simulink model "Book6331"  (R2019b)
settings: Solver=ode4  StartTime=0.0  StopTime=10.0  FixedStep=0.001  RelTol=1e-3
settings Model: Creator=user  LastModifiedBy=user

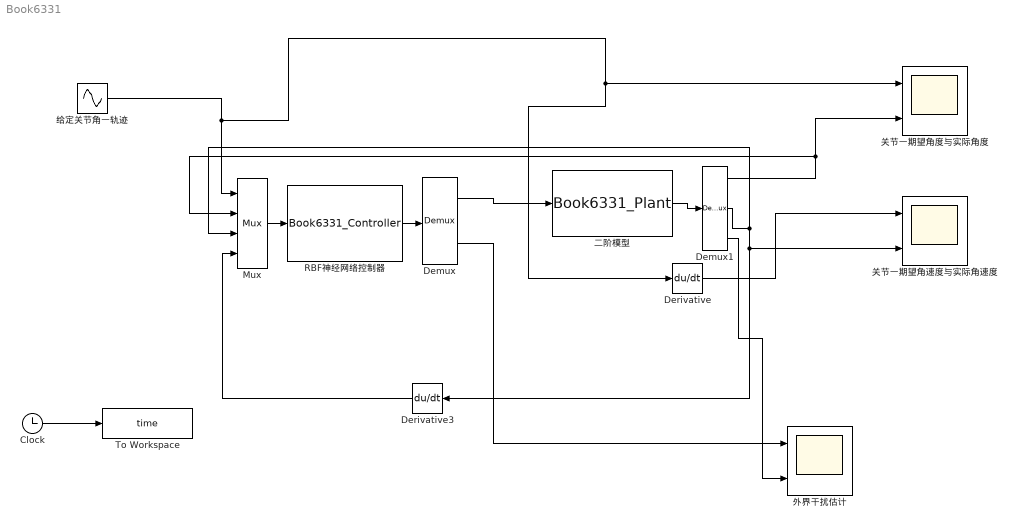
== system Book6331 ==
  Clock : Clock
  Demux : Demux  Outputs=2
  Demux1 : Demux  Outputs=3
  Derivative : Derivative
  Derivative3 : Derivative
  Mux : Mux
  RBF神经网络控制器 : S-Function  FunctionName=Book6331_Controller  SFunctionDeploymentMode=off  EnableBusSupport=off
  To Workspace : ToWorkspace  VariableName=time  SaveFormat=Timeseries  SampleTime=-1
  二阶模型 : S-Function  FunctionName=Book6331_Plant  SFunctionDeploymentMode=off  EnableBusSupport=off
  关节一期望角度与实际角度 : Scope  NumInputPorts=2
  关节一期望角速度与实际角速度 : Scope  NumInputPorts=2
  外界干扰估计 : Scope  NumInputPorts=2
  给定关节角一轨迹 : Sin  SampleTime=0
  wires:
  二阶模型/1 -> Demux1/1
  Derivative/1 -> 关节一期望角速度与实际角速度/1
  给定关节角一轨迹/1 -> Derivative/1, 关节一期望角度与实际角度/1, Mux/1
  RBF神经网络控制器/1 -> Demux/1
  Mux/1 -> RBF神经网络控制器/1
  Derivative3/1 -> Mux/4
  Demux1/2 -> Mux/3, Derivative3/1, 关节一期望角速度与实际角速度/2
  Demux/2 -> 外界干扰估计/1
  Demux/1 -> 二阶模型/1
  Clock/1 -> To Workspace/1
  Demux1/1 -> Mux/2, 关节一期望角度与实际角度/2
  Demux1/3 -> 外界干扰估计/2
